simulink model "controller_arduino"  (R2022b)
settings: Solver=FixedStepDiscrete  StartTime=0.0  StopTime=10.0  FixedStep=1/10  RelTol=1e-3  EnableMultiTasking=on
undefined symbols (not defined in the file): MAX_SPEED_BACKWARD, MAX_SPEED_FORWARD
libraries: arduinolib x18, simulink x1
settings Model: ExtModeTrigDuration=2  Creator=DAUIN-Win10  LastModifiedBy=Pietro
settings OptimizationCC: EnhancedBackFolding=on  PassReuseOutputArgsAs=Individual arguments  ZeroExternalMemoryAtStartup=off  ZeroInternalMemoryAtStartup=off  MaxStackSize=64  OptimizeBlockOrder=speed  DifferentSizesBufferReuse=on  OptimizationCustomize=off  EfficientTunableParamExpr=on
settings DebuggingCC: ParameterTunabilityLossMsg=error  UnconnectedInputMsg=warning  UnconnectedOutputMsg=warning  UnconnectedLineMsg=warning
settings HardwareCC: ProdBitPerInt=16  ProdBitPerPointer=16  ProdBitPerSizeT=16  ProdBitPerPtrDiffT=16  ProdLargestAtomicFloat=None  ProdWordSize=8  ProdHWDeviceType=Atmel->AVR
settings ModelReferenceCC: EnableRefExpFcnMdlSchedulingChecks=on
settings SFSimCC: MATLABDynamicMemAlloc=off
settings RTWCC: Description=Embedded Coder  SystemTargetFile=ert.tlc  HardwareBoard=Arduino Uno  TLCOptions=-aInlineSetEventsForThisBaseRateFcn=TLC_FALSE -aSuppressMultiTaskScheduler=TLC_FALSE -aRateBasedStepFcn=1  TemplateMakefile=ert_default_tmf  Toolchain=Arduino AVR  BuildConfiguration=Faster Runs  DLArmComputeVersion=19.05
settings CodeAppCC: ForceParamTrailComments=on  IgnoreCustomStorageClasses=off  OperatorAnnotations=on  SimulinkDataObjDesc=on  SFDataObjDesc=on  InsertBlockDesc=on
settings ERTTargetCC: SupportContinuousTime=on  SupportVariableSizeSignals=on  ExtModeTransport=3  ExtModeStaticAlloc=on  ExtModeStaticAllocSize=250  ExtModeMexFile=ext_xcp  ExtModeIntrfLevel=Level2 - Open

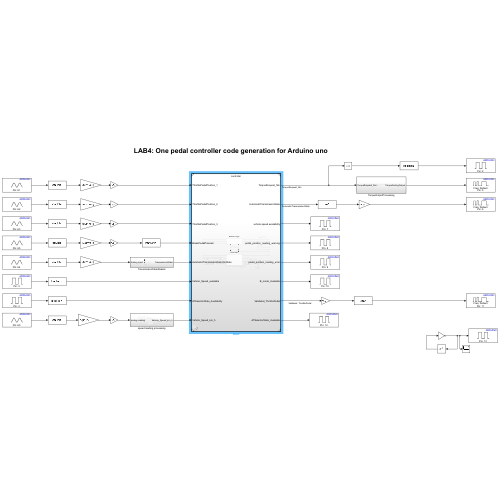
[thumbnail: Simulink's stored preview of the top-level diagram]
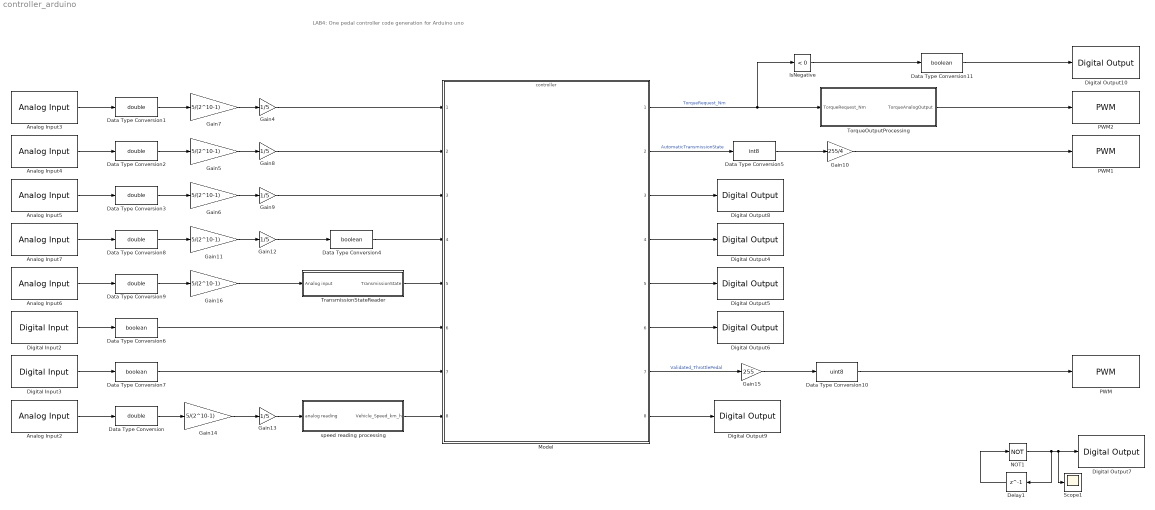
== system controller_arduino ==
  note: LAB4: One pedal controller code generation for Arduino uno
  Analog Input2 : arduinolib/Analog Input  pinNumber=0  ReadResultsOnly=off  ConversionTriggerSource=Software  ExternalTriggerType=uint32( 0 )  OutputDataType=uint16  EnableConversionCompleteNotify=off  EnableOuputStatus=off  SampleTime=-1  blockPlatform=arduino
  Analog Input3 : arduinolib/Analog Input  pinNumber=1  ReadResultsOnly=off  ConversionTriggerSource=Software  ExternalTriggerType=uint32( 0 )  OutputDataType=uint16  EnableConversionCompleteNotify=off  EnableOuputStatus=off  SampleTime=-1  blockPlatform=arduino
  Analog Input4 : arduinolib/Analog Input  pinNumber=2  ReadResultsOnly=off  ConversionTriggerSource=Software  ExternalTriggerType=uint32( 0 )  OutputDataType=uint16  EnableConversionCompleteNotify=off  EnableOuputStatus=off  SampleTime=-1  blockPlatform=arduino
  Analog Input5 : arduinolib/Analog Input  pinNumber=3  ReadResultsOnly=off  ConversionTriggerSource=Software  ExternalTriggerType=uint32( 0 )  OutputDataType=uint16  EnableConversionCompleteNotify=off  EnableOuputStatus=off  SampleTime=-1  blockPlatform=arduino
  Analog Input6 : arduinolib/Analog Input  pinNumber=4  ReadResultsOnly=off  ConversionTriggerSource=Software  ExternalTriggerType=uint32( 0 )  OutputDataType=uint16  EnableConversionCompleteNotify=off  EnableOuputStatus=off  SampleTime=-1  blockPlatform=arduino
  Analog Input7 : arduinolib/Analog Input  pinNumber=5  ReadResultsOnly=off  ConversionTriggerSource=Software  ExternalTriggerType=uint32( 0 )  OutputDataType=uint16  EnableConversionCompleteNotify=off  EnableOuputStatus=off  SampleTime=-1  blockPlatform=arduino
  Data Type Conversion{,1..3,8..9} (6 alike) : DataTypeConversion  OutDataTypeStr=double  SaturateOnIntegerOverflow=off  RndMeth=Floor
  Data Type Conversion10 : DataTypeConversion  OutDataTypeStr=uint8  SaturateOnIntegerOverflow=off  RndMeth=Floor
  Data Type Conversion{4,6..7,11} (4 alike) : DataTypeConversion  OutDataTypeStr=boolean  SaturateOnIntegerOverflow=off  RndMeth=Floor
  Data Type Conversion5 : DataTypeConversion  OutDataTypeStr=int8  SaturateOnIntegerOverflow=off  RndMeth=Floor
  Delay1 : Delay  DelayLength=1  SampleTime=0.5
  Digital Input2 : arduinolib/Digital Input  pinNumber=3  mode=Default  Direction=input  SampleTime=-1  blockPlatform=arduino
  Digital Input3 : arduinolib/Digital Input  pinNumber=4  mode=Default  Direction=input  SampleTime=-1  blockPlatform=arduino
  Digital Output10 : arduinolib/Digital Output  pinNumber=2  Direction=output  blockPlatform=arduino
  Digital Output4 : arduinolib/Digital Output  pinNumber=8  Direction=output  blockPlatform=arduino
  Digital Output5 : arduinolib/Digital Output  pinNumber=9  Direction=output  blockPlatform=arduino
  Digital Output6 : arduinolib/Digital Output  pinNumber=10  Direction=output  blockPlatform=arduino
  Digital Output7 : arduinolib/Digital Output  pinNumber=13  Direction=output  blockPlatform=arduino
  Digital Output8 : arduinolib/Digital Output  pinNumber=7  Direction=output  blockPlatform=arduino
  Digital Output9 : arduinolib/Digital Output  pinNumber=12  Direction=output  blockPlatform=arduino
  Gain10 : Gain  Gain=255/4
  Gain{5..7,11,14,16} (6 alike) : Gain  Gain=5/(2^10-1)
  Gain{4,8..9,12..13} (5 alike) : Gain  Gain=1/5
  Gain15 : Gain  Gain=255
  IsNegative : simulink/Logic and Bit Operations/Compare To Zero  relop=<  OutDataTypeStr=boolean
      settings: LibrarySourceBlock=|
      | simulink/Quick Insert/Logic and Bit
      | Operations/IsNegative
  Model : ModelReference  ModelNameDialog=controller  SimulationMode=Normal  ModelReferenceVersion=3.6
  NOT1 : Logic  Operator=NOT  IconShape=distinctive  AllPortsSameDT=off  OutDataTypeStr=boolean
  PWM : arduinolib/PWM  pinNumber=11  frequencyType=Default  desiredFrequency=490.2  achievableFrequency=490.2
  PWM1 : arduinolib/PWM  pinNumber=6  frequencyType=Default  desiredFrequency=490.2  achievableFrequency=490.2
  PWM2 : arduinolib/PWM  pinNumber=5  frequencyType=Default  desiredFrequency=490.2  achievableFrequency=490.2
  Scope1 : Scope
  TorqueOutputProcessing : Subsystem
  TransmissionStateReader : Subsystem
  speed reading processing : Subsystem
  wires:
  Model/3 -> Digital Output8/1
  Data Type Conversion2/1 -> Gain5/1
  Analog Input5/1 -> Data Type Conversion3/1
  Data Type Conversion11/1 -> Digital Output10/1
  Analog Input2/1 -> Data Type Conversion/1
  Data Type Conversion9/1 -> Gain16/1
  Gain5/1 -> Gain8/1
  Gain11/1 -> Gain12/1
  Gain15/1 -> Data Type Conversion10/1
  Analog Input7/1 -> Data Type Conversion8/1
  Gain4/1 -> Model/1
  speed reading processing/1(Vehicle_Speed_km_h) -> Model/8
  Model/6 -> Digital Output6/1
  Data Type Conversion5/1 -> Gain10/1
  Gain13/1 -> speed reading processing/1(analog reading)
  Data Type Conversion3/1 -> Gain6/1
  Data Type Conversion/1 -> Gain14/1
  Gain16/1 -> TransmissionStateReader/1(Analog input)
  Model/1 -> IsNegative/1, TorqueOutputProcessing/1(TorqueRequest_Nm)  "TorqueRequest_Nm"
  Gain12/1 -> Data Type Conversion4/1
  Analog Input6/1 -> Data Type Conversion9/1
  Gain9/1 -> Model/3
  Model/8 -> Digital Output9/1
  Model/7 -> Gain15/1  "Validated_ThrottlePedal"
  TorqueOutputProcessing/1(TorqueAnalogOutput) -> PWM2/1
  Gain8/1 -> Model/2
  Data Type Conversion1/1 -> Gain7/1
  Data Type Conversion7/1 -> Model/7
  Model/2 -> Data Type Conversion5/1  "AutomaticTransmissionState"
  Digital Input3/1 -> Data Type Conversion7/1
  Digital Input2/1 -> Data Type Conversion6/1
  Data Type Conversion6/1 -> Model/6
  Analog Input3/1 -> Data Type Conversion1/1
  Data Type Conversion8/1 -> Gain11/1
  Analog Input4/1 -> Data Type Conversion2/1
  Delay1/1 -> NOT1/1
  IsNegative/1 -> Data Type Conversion11/1
  Data Type Conversion4/1 -> Model/4
  Model/4 -> Digital Output4/1
  NOT1/1 -> Delay1/1, Scope1/1, Digital Output7/1
  Gain7/1 -> Gain4/1
  Gain6/1 -> Gain9/1
  Gain10/1 -> PWM1/1
  Gain14/1 -> Gain13/1
  Data Type Conversion10/1 -> PWM/1
  TransmissionStateReader/1(TransmissionState) -> Model/5
  Model/5 -> Digital Output5/1

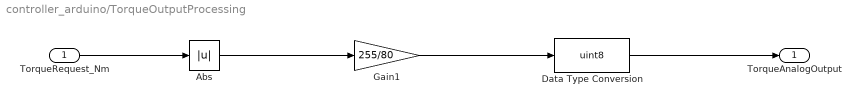
== system controller_arduino/TorqueOutputProcessing ==
  TorqueRequest_Nm : Inport
  Abs : Abs  SaturateOnIntegerOverflow=off
  Data Type Conversion : DataTypeConversion  OutDataTypeStr=uint8  SaturateOnIntegerOverflow=off  RndMeth=Floor
  Gain1 : Gain  Gain=255/80
  TorqueAnalogOutput : Outport
  wires:
  Gain1/1 -> Data Type Conversion/1
  Data Type Conversion/1 -> TorqueAnalogOutput/1
  TorqueRequest_Nm/1 -> Abs/1
  Abs/1 -> Gain1/1

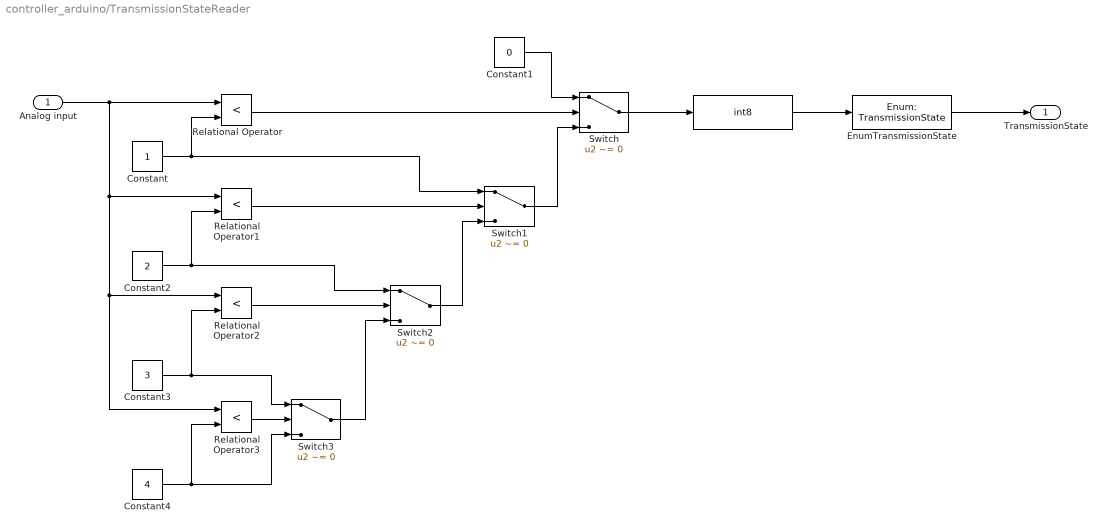
== system controller_arduino/TransmissionStateReader ==
  Analog input : Inport
  " " : DataTypeConversion  OutDataTypeStr=int8  SaturateOnIntegerOverflow=off  RndMeth=Floor
  Constant : Constant
  Constant1 : Constant  Value=0
  Constant2 : Constant  Value=2
  Constant3 : Constant  Value=3
  Constant4 : Constant  Value=4
  EnumTransmissionState : DataTypeConversion  OutDataTypeStr=Enum: TransmissionState  SaturateOnIntegerOverflow=off  RndMeth=Floor
  Relational Operator{,1..3} (4 alike) : RelationalOperator  Operator=<  OutDataTypeStr=boolean  RndMeth=Simplest  InputSameDT=off
  Switch{,1..3} (4 alike) : Switch  Criteria=u2 ~= 0  SaturateOnIntegerOverflow=off  InputSameDT=off
  TransmissionState : Outport
  wires:
  EnumTransmissionState/1 -> TransmissionState/1
  Switch/1 -> " "/1
  Analog input/1 -> Relational Operator3/1, Relational Operator2/1, Relational Operator1/1, Relational Operator/1
  Constant/1 -> Relational Operator/2, Switch1/1
  Relational Operator/1 -> Switch/2
  Constant1/1 -> Switch/1
  Constant2/1 -> Relational Operator1/2, Switch2/1
  Switch1/1 -> Switch/3
  Relational Operator1/1 -> Switch1/2
  Relational Operator2/1 -> Switch2/2
  Switch2/1 -> Switch1/3
  Constant3/1 -> Switch3/1, Relational Operator2/2
  Switch3/1 -> Switch2/3
  Relational Operator3/1 -> Switch3/2
  Constant4/1 -> Switch3/3, Relational Operator3/2
  " "/1 -> EnumTransmissionState/1

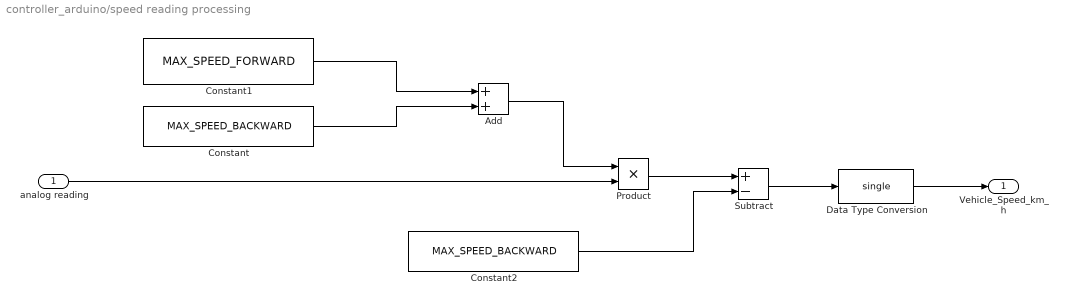
== system controller_arduino/speed reading processing ==
  analog reading : Inport
  Add : Sum
  Constant : Constant  Value=MAX_SPEED_BACKWARD
  Constant1 : Constant  Value=MAX_SPEED_FORWARD
  Constant2 : Constant  Value=MAX_SPEED_BACKWARD
  Data Type Conversion : DataTypeConversion  OutDataTypeStr=single  SaturateOnIntegerOverflow=off  RndMeth=Floor
  Product : Product
  Subtract : Sum  Inputs=+-
  Vehicle_Speed_km_h : Outport
  wires:
  Constant/1 -> Add/2
  Constant1/1 -> Add/1
  Add/1 -> Product/1
  Product/1 -> Subtract/1
  Constant2/1 -> Subtract/2
  Subtract/1 -> Data Type Conversion/1
  analog reading/1 -> Product/2
  Data Type Conversion/1 -> Vehicle_Speed_km_h/1
